simulink model "PMSM"  (R2024b)
settings: Solver=VariableStepAuto  StartTime=0.0  StopTime=1  RelTol=1e-3
settings Model: Creator=Ahmad  LastModifiedBy=Ahmad

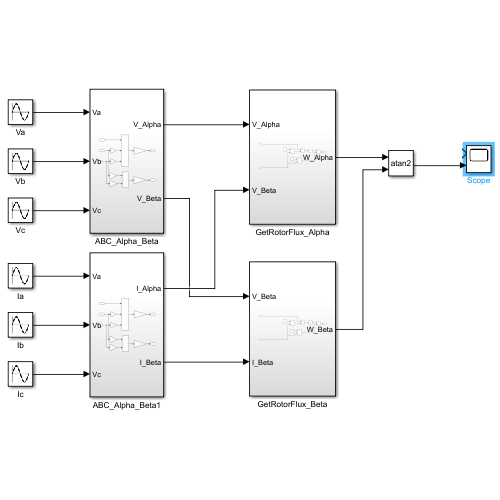
[thumbnail: Simulink's stored preview of the top-level diagram]
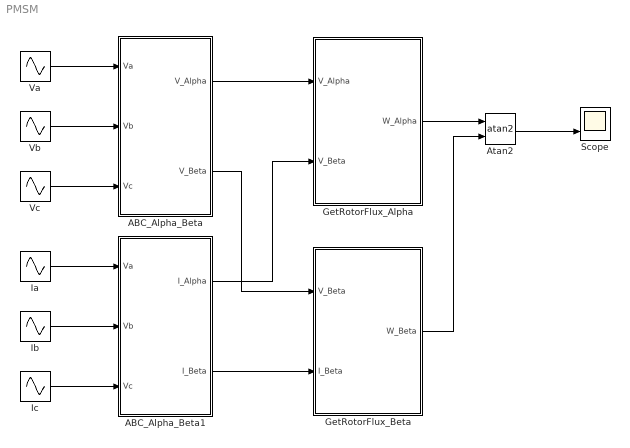
== system PMSM ==
  ABC_Alpha_Beta : Subsystem
  ABC_Alpha_Beta1 : Subsystem
  Atan2 : Trigonometry  Operator=atan2
  GetRotorFlux_Alpha : Subsystem
  GetRotorFlux_Beta : Subsystem
  Ia : Sin  Amplitude=2  Frequency=300  SampleTime=0
  Ib : Sin  Amplitude=2  Frequency=300  Phase=-120*(pi/180)  SampleTime=0
  Ic : Sin  Amplitude=2  Frequency=300  Phase=120*(pi/180)  SampleTime=0
  Scope : Scope  NumInputPorts=2
  Va : Sin  Amplitude=12  Frequency=300  SampleTime=0
  Vb : Sin  Amplitude=12  Frequency=300  Phase=-120*(pi/180)  SampleTime=0
  Vc : Sin  Amplitude=12  Frequency=300  Phase=120*(pi/180)  SampleTime=0
  wires:
  Va/1 -> ABC_Alpha_Beta/1(Va)
  Vb/1 -> ABC_Alpha_Beta/2(Vb)
  Vc/1 -> ABC_Alpha_Beta/3(Vc)
  Ic/1 -> ABC_Alpha_Beta1/3(Vc)
  Ib/1 -> ABC_Alpha_Beta1/2(Vb)
  Ia/1 -> ABC_Alpha_Beta1/1(Va)
  ABC_Alpha_Beta/1(V_Alpha) -> GetRotorFlux_Alpha/1(V_Alpha)
  ABC_Alpha_Beta1/1(I_Alpha) -> GetRotorFlux_Alpha/2(V_Beta)
  ABC_Alpha_Beta/2(V_Beta) -> GetRotorFlux_Beta/1(V_Beta)
  ABC_Alpha_Beta1/2(I_Beta) -> GetRotorFlux_Beta/2(I_Beta)
  GetRotorFlux_Alpha/1(W_Alpha) -> Atan2/1
  GetRotorFlux_Beta/1(W_Beta) -> Atan2/2
  Atan2/1 -> Scope/2

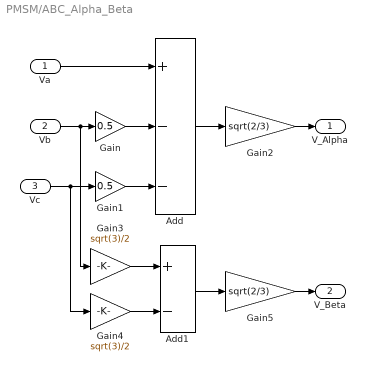
== system PMSM/ABC_Alpha_Beta ==
  Va : Inport
  Vb : Inport  Port=2
  Vc : Inport  Port=3
  Add : Sum  Inputs=+--
  Add1 : Sum  Inputs=+-
  Gain : Gain  Gain=0.5
  Gain1 : Gain  Gain=0.5
  Gain2 : Gain  Gain=sqrt(2/3)
  Gain3 : Gain  Gain=sqrt(3)/2
  Gain4 : Gain  Gain=sqrt(3)/2
  Gain5 : Gain  Gain=sqrt(2/3)
  V_Alpha : Outport
  V_Beta : Outport  Port=2
  wires:
  Vb/1 -> Gain3/1, Gain/1
  Gain4/1 -> Add1/2
  Gain/1 -> Add/2
  Gain3/1 -> Add1/1
  Vc/1 -> Gain4/1, Gain1/1
  Add/1 -> Gain2/1
  Add1/1 -> Gain5/1
  Gain1/1 -> Add/3
  Va/1 -> Add/1
  Gain2/1 -> V_Alpha/1
  Gain5/1 -> V_Beta/1

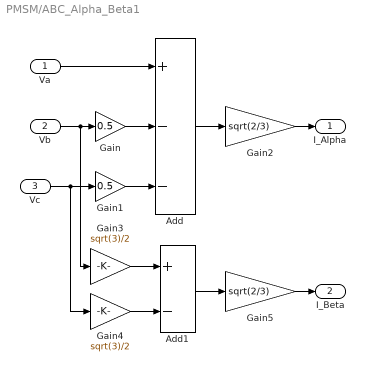
== system PMSM/ABC_Alpha_Beta1 ==
  Va : Inport
  Vb : Inport  Port=2
  Vc : Inport  Port=3
  Add : Sum  Inputs=+--
  Add1 : Sum  Inputs=+-
  Gain : Gain  Gain=0.5
  Gain1 : Gain  Gain=0.5
  Gain2 : Gain  Gain=sqrt(2/3)
  Gain3 : Gain  Gain=sqrt(3)/2
  Gain4 : Gain  Gain=sqrt(3)/2
  Gain5 : Gain  Gain=sqrt(2/3)
  I_Alpha : Outport
  I_Beta : Outport  Port=2
  wires:
  Vb/1 -> Gain3/1, Gain/1
  Gain4/1 -> Add1/2
  Gain/1 -> Add/2
  Gain3/1 -> Add1/1
  Vc/1 -> Gain4/1, Gain1/1
  Add/1 -> Gain2/1
  Add1/1 -> Gain5/1
  Gain1/1 -> Add/3
  Va/1 -> Add/1
  Gain2/1 -> I_Alpha/1
  Gain5/1 -> I_Beta/1

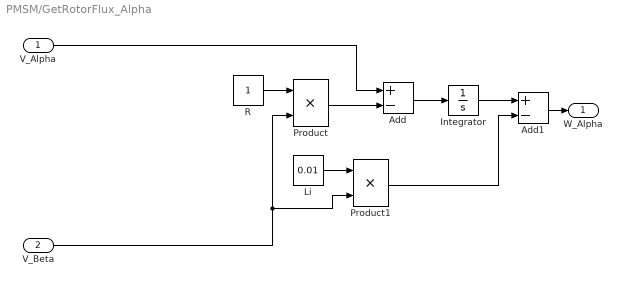
== system PMSM/GetRotorFlux_Alpha ==
  V_Alpha : Inport
  V_Beta : Inport  Port=2
  Add : Sum  Inputs=+-
  Add1 : Sum  Inputs=+-
  Integrator : Integrator
  Li : Constant  Value=0.01
  Product : Product
  Product1 : Product
  R : Constant
  W_Alpha : Outport
  wires:
  V_Alpha/1 -> Add/1
  R/1 -> Product/1
  Li/1 -> Product1/1
  Product/1 -> Add/2
  Product1/1 -> Add1/2
  Add/1 -> Integrator/1
  Integrator/1 -> Add1/1
  V_Beta/1 -> Product1/2, Product/2
  Add1/1 -> W_Alpha/1

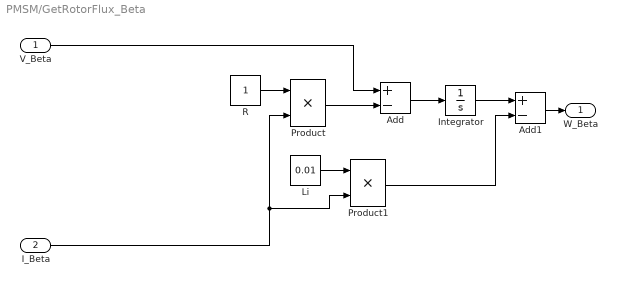
== system PMSM/GetRotorFlux_Beta ==
  V_Beta : Inport
  I_Beta : Inport  Port=2
  Add : Sum  Inputs=+-
  Add1 : Sum  Inputs=+-
  Integrator : Integrator
  Li : Constant  Value=0.01
  Product : Product
  Product1 : Product
  R : Constant
  W_Beta : Outport
  wires:
  V_Beta/1 -> Add/1
  R/1 -> Product/1
  Li/1 -> Product1/1
  Product/1 -> Add/2
  Product1/1 -> Add1/2
  Add/1 -> Integrator/1
  Integrator/1 -> Add1/1
  I_Beta/1 -> Product1/2, Product/2
  Add1/1 -> W_Beta/1
